simulink model "ex21"  (R2014a)
settings: Solver=ode45  StartTime=0.0  StopTime=100.0  RelTol=1e-3
settings Model: Creator=liang  LastModifiedBy=liang

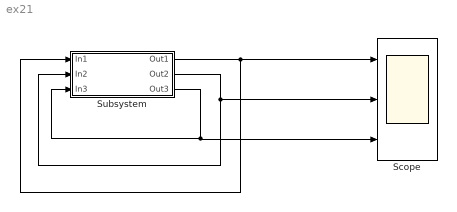
== system ex21 ==
  Scope : Scope  NumInputPorts=3
      settings: YMin=-5~-5~-5  YMax=5~5~5  MaxDataPoints=50000
  Subsystem : Subsystem
  wires:
  Subsystem/1(Out1) -> Scope/1, Subsystem/1(In1)
  Subsystem/3(Out3) -> Scope/3, Subsystem/3(In3)
  Subsystem/2(Out2) -> Scope/2, Subsystem/2(In2)

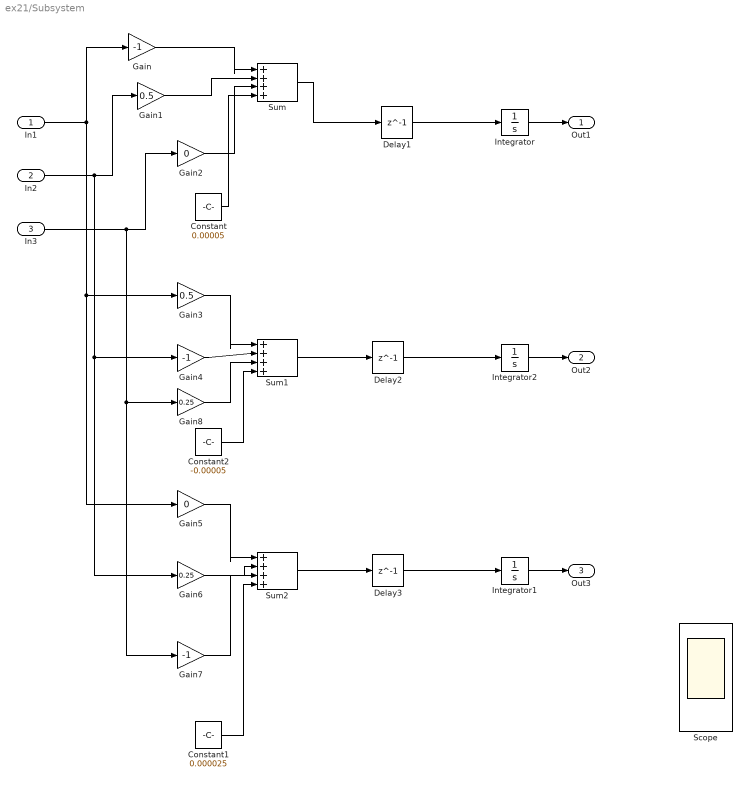
== system ex21/Subsystem ==
  In1 : Inport
  In2 : Inport  Port=2
  In3 : Inport  Port=3
  Constant : Constant  Value=0.00005
  Constant1 : Constant  Value=0.000025
  Constant2 : Constant  Value=-0.00005
  Delay1 : Delay  DelayLength=1  SampleTime=0.01
  Delay2 : Delay  DelayLength=1  SampleTime=0.01
  Delay3 : Delay  DelayLength=1  SampleTime=0.01
  Gain : Gain  Gain=-1
  Gain1 : Gain  Gain=0.5
  Gain2 : Gain  Gain=0
  Gain3 : Gain  Gain=0.5
  Gain4 : Gain  Gain=-1
  Gain5 : Gain  Gain=0
  Gain6 : Gain  Gain=0.25
  Gain7 : Gain  Gain=-1
  Gain8 : Gain  Gain=0.25
  Integrator : Integrator  InitialCondition=-11.3636
  Integrator1 : Integrator  InitialCondition=-8.1818
  Integrator2 : Integrator  InitialCondition=-32.7272
  Scope : Scope
  Sum : Sum  Inputs=|++++
  Sum1 : Sum  Inputs=|++++
  Sum2 : Sum  Inputs=|++++
  Out1 : Outport
  Out2 : Outport  Port=2
  Out3 : Outport  Port=3
  wires:
  Integrator/1 -> Out1/1
  Integrator2/1 -> Out2/1
  Integrator1/1 -> Out3/1
  Sum/1 -> Delay1/1
  In1/1 -> Gain5/1, Gain3/1, Gain/1
  Gain/1 -> Sum/1
  In2/1 -> Gain6/1, Gain4/1, Gain1/1
  Gain1/1 -> Sum/2
  In3/1 -> Gain8/1, Gain7/1, Gain2/1
  Gain2/1 -> Sum/3
  Sum1/1 -> Delay2/1
  Gain3/1 -> Sum1/1
  Gain4/1 -> Sum1/2
  Gain5/1 -> Sum2/1
  Gain6/1 -> Sum2/2
  Gain7/1 -> Sum2/3
  Sum2/1 -> Delay3/1
  Delay1/1 -> Integrator/1
  Delay2/1 -> Integrator2/1
  Delay3/1 -> Integrator1/1
  Constant/1 -> Sum/4
  Constant1/1 -> Sum2/4
  Gain8/1 -> Sum1/3
  Constant2/1 -> Sum1/4
